simulink model "obstacleStopper"  (R2016a)
settings: Solver=FixedStepAuto  StartTime=0.0  StopTime=inf  FixedStep=0.02  RelTol=1e-3
undefined symbols (not defined in the file): Angular, Linear
libraries: robotlib x4
settings Model: Creator=sprinkle  LastModifiedBy=sprinkle
settings OptimizationCC: OptimizeModelRefInitCode=on  LifeSpan=Inf  MaxStackSize=64
settings HardwareCC: ProdBitPerPointer=32  ProdLargestAtomicFloat=None  ProdIntDivRoundTo=Undefined  ProdEndianess=Unspecified  ProdWordSize=32  ProdHWDeviceType=Generic->Unspecified (assume 32-bit Generic)
settings RTWCC: SystemTargetFile=ert.tlc  HardwareBoard=Robot Operating System (ROS)  TemplateMakefile=ert_default_tmf  GenerateReport=on  Toolchain=Catkin  IncludeHyperlinkInReport=on  LaunchReport=on  TargetLang=C++  GenerateTraceInfo=on  GenerateTraceReport=on  GenerateTraceReportSl=on  GenerateTraceReportSf=on  GenerateTraceReportEml=on
settings CodeAppCC: ForceParamTrailComments=on  IgnoreCustomStorageClasses=off  OperatorAnnotations=on  SimulinkDataObjDesc=on  SFDataObjDesc=on  MATLABFcnDesc=on  InsertBlockDesc=on  MATLABSourceComments=on

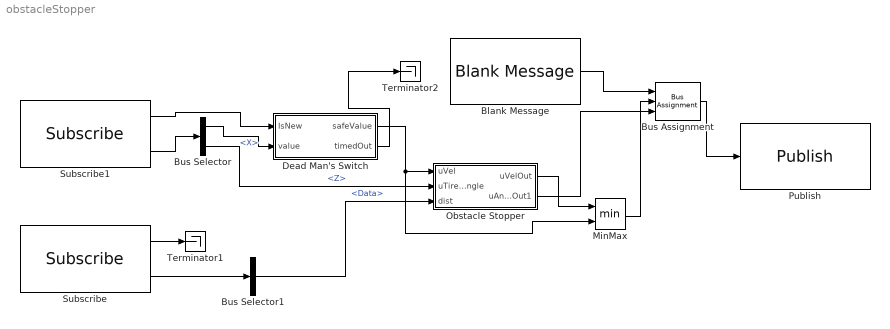
== system obstacleStopper ==
  Blank Message : robotlib/Blank Message  SourceLibraryInfo=This block requires Robotics System Toolbox  messageType=geometry_msgs/Twist  SampleTime=inf
  Bus Assignment : BusAssignment  AssignedSignals=Linear.X,Angular.Z
  Bus Selector : BusSelector  OutputSignals=Linear.X,Angular.Z
  Bus Selector1 : BusSelector  OutputSignals=Data
  Dead Man's Switch : Subsystem  TreatAsAtomicUnit=on  mask{stepSize=0.02, timeout=0.2}
      mask prompts: stepSize "Simulation step size"; timeout "Timeout (in seconds)"
      mask help: Interprets whether a new message has been recently received, and if so permits the data in 'value' to be passed through. Otherwise, 0 is outputted from 'safeValue'
      mask Help: Interprets whether a new message has been recently received, and if so permits the data in 'value' to be passed through. Otherwise, 0 is outputted from 'safeValue'
  MinMax : MinMax  Inputs=2
  Obstacle Stopper : Subsystem
  Publish : robotlib/Publish  SourceLibraryInfo=This block requires Robotics System Toolbox  topicSource=Specify your own  topic=/catvehicle/cmd_vel_safe  messageType=geometry_msgs/Twist  messageQueueLength=1
  Subscribe : robotlib/Subscribe  SourceLibraryInfo=This block requires Robotics System Toolbox  topicSource=Select from ROS network  topic=/catvehicle/distanceEstimator/dist  messageType=std_msgs/Float32  sampleTime=-1  messageQueueLength=1
  Subscribe1 : robotlib/Subscribe  SourceLibraryInfo=This block requires Robotics System Toolbox  topicSource=Specify your own  topic=/catvehicle/cmd_vel  messageType=geometry_msgs/Twist  sampleTime=-1  messageQueueLength=1
  Terminator1 : Terminator
  Terminator2 : Terminator
  wires:
  Subscribe1/2 -> Bus Selector/1
  Subscribe1/1 -> Dead Man's Switch/1(IsNew)
  Bus Selector/2 -> Obstacle Stopper/2(uTireAngle)  "<Z>"
  Blank Message/1 -> Bus Assignment/1
  Bus Assignment/1 -> Publish/1
  Obstacle Stopper/2(uAngleOut1) -> Bus Assignment/3
  Subscribe/1 -> Terminator1/1
  Subscribe/2 -> Bus Selector1/1
  Bus Selector1/1 -> Obstacle Stopper/3(dist)  "<Data>"
  Dead Man's Switch/1(safeValue) -> MinMax/2, Obstacle Stopper/1(uVel)
  Bus Selector/1 -> Dead Man's Switch/2(value)  "<X>"
  Dead Man's Switch/2(timedOut) -> Terminator2/1
  MinMax/1 -> Bus Assignment/2
  Obstacle Stopper/1(uVelOut) -> MinMax/1

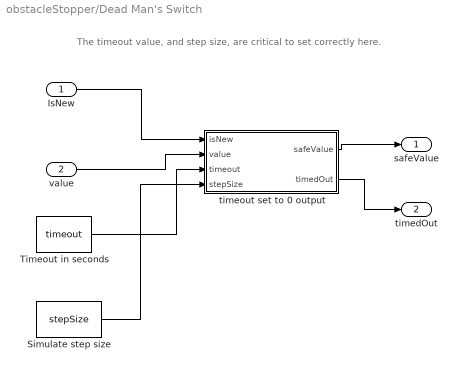
== system obstacleStopper/Dead Man's Switch ==
  note: The timeout value, and step size, are critical to set correctly here.
  IsNew : Inport
  value : Inport  Port=2
  Simulate step size : Constant  Value=stepSize
  Timeout in seconds : Constant  Value=timeout
  timeout set to 0 output : MATLAB Function  TreatAsAtomicUnit=on
  safeValue : Outport  InitialOutput=[0]
  timedOut : Outport  Port=2  InitialOutput=[0]
  wires:
  IsNew/1 -> timeout set to 0 output/1(isNew)
  timeout set to 0 output/1(safeValue) -> safeValue/1
  value/1 -> timeout set to 0 output/2(value)
  Timeout in seconds/1 -> timeout set to 0 output/3(timeout)
  timeout set to 0 output/2(timedOut) -> timedOut/1
  Simulate step size/1 -> timeout set to 0 output/4(stepSize)

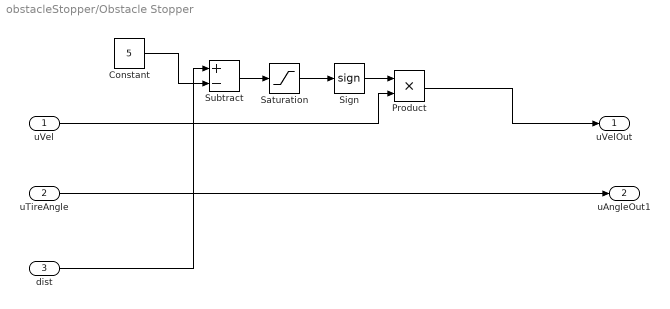
== system obstacleStopper/Obstacle Stopper ==
  uVel : Inport
  uTireAngle : Inport  Port=2
  dist : Inport  Port=3
  Constant : Constant  Value=5
  Product : Product
  Saturation : Saturate  UpperLimit=1  LowerLimit=0
  Sign : Signum
  Subtract : Sum  Inputs=+-
  uVelOut : Outport
  uAngleOut1 : Outport  Port=2
  wires:
  Constant/1 -> Subtract/2
  dist/1 -> Subtract/1
  Subtract/1 -> Saturation/1
  Saturation/1 -> Sign/1
  uVel/1 -> Product/2
  Sign/1 -> Product/1
  Product/1 -> uVelOut/1
  uTireAngle/1 -> uAngleOut1/1

== matlab function obstacleStopper/Dead Man's Switch/timeout set to 0 output ==
  data: isNew input; safeValue output; value input; timeout input; timedOut output; stepSize input
function [safeValue,timedOut] = fcn(isNew,value,timeout,stepSize)
%#codegen
persistent sinceLastMsg
timedOut=true;
if isempty(sinceLastMsg)
    sinceLastMsg=(timeout/stepSize)+1;
end

safeValue=0;
% if no new message
% after timeout, we output 0
if( isNew == true )
    sinceLastMsg = 0;
else
    sinceLastMsg = sinceLastMsg+1;
end

% Note: we require step size as an input here, and depend on our
% system being executed at a regular rate, or bad things will happen
if( sinceLastMsg < timeout/stepSize )
    timedOut = false;
end
    
if( timedOut == false )
    safeValue = value;
end
